simulink model "Lab_9_Electric_Power_Steering"  (R2023b)
settings: Solver=VariableStepAuto  StartTime=0.0  StopTime=20  RelTol=1e-3
libraries: fl_lib x20, nesl_utility x7, ee_lib x2, simulink x1
settings Model: Creator=AHMED MOHSEN  LastModifiedBy=AHMED MOHSEN

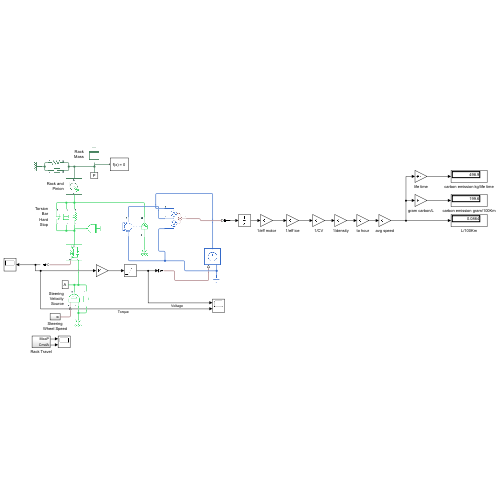
[thumbnail: Simulink's stored preview of the top-level diagram]
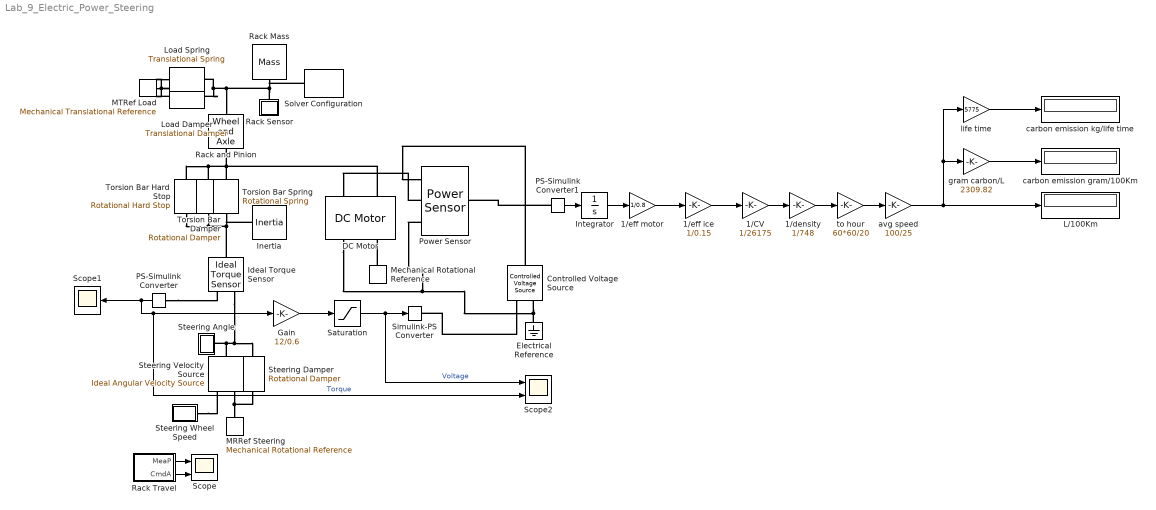
== system Lab_9_Electric_Power_Steering ==
  1/CV : Gain  Gain=1/26175
  1/density : Gain  Gain=1/748
  1/eff ice : Gain  Gain=1/0.15
  1/eff motor : Gain  Gain=1/0.8
  Controlled Voltage Source : fl_lib/Electrical/Electrical Sources/Controlled Voltage Source
  DC Motor : ee_lib/Electromechanical/Brushed Motors/DC Motor  field_option=ee.enum.field_option.pm  Rf=100 Ohm  Lf=1 H  Laf=0.15 H  If0=0 A  parameterization=ee.enum.dcparam_option.circuit_param  Ra=3.9 Ohm  La=12e-6 H  emf_or_torque=ee.enum.emf_or_torque.kv  Kv=0.072e-3 V/rpm  Ki=6.876e-4 N*m/A  T_stall=0.24e-3 N*m  w_max=19100 rpm  w_rated=15000 rpm  P_rated=0.08 W  V_rated=1.5 V  lam_param=ee.enum.lam_param.damping  i_noload=0 A  V_i_noload=1.5 V  J=0.01 cm^2*g  lam=0 N*m*s/rad  speed0=0 rpm  enable_fault_armature=simscape.enum.onoff.off  rev_faulted=1 / 3  G_faulted_armature=1e-5 S  fault_trigger_armature=ee.enum.faults.faultTrigger.temporal  t_fault_armature=1 s  max_permissible_current_armature=inf A  t_fail_on_current_armature=1 s  enable_fault_field=simscape.enum.onoff.off  G_faulted_field=1e-5 S  fault_trigger_field=ee.enum.faults.faultTrigger.temporal  t_fault_field=1 s  max_permissible_current_field=inf A  t_fail_on_current_field=1 s  fault_action=simscape.enum.assert.action.none  alpha=3.93e-3 1/K  Tmeas=25 degC  thermal_mass=100 J/K  initial_temperature=25 degC
  Electrical Reference : fl_lib/Electrical/Electrical Elements/Electrical Reference
  Gain : Gain  Gain=12/0.6
  Ideal Torque Sensor : fl_lib/Mechanical/Mechanical Sensors/Ideal Torque Sensor
  Inertia : fl_lib/Mechanical/Rotational Elements/Inertia  inertia=0.01 kg*m^2  num_ports=foundation.enum.numPorts2.one  w_specify=off  w_priority=High  w=0 rad/s  w_nominal_specify=off  w_nominal_unit=rad/s  w_nominal_value=1  t_specify=off  t_priority=None  t=0 N*m  t_nominal_specify=off  t_nominal_unit=N*m  t_nominal_value=1
  Integrator : Integrator
  L/100Km : Display
  Load Damper : fl_lib/Mechanical/Translational Elements/Translational Damper  Tag=Factory Generic  D=284 N/(m/s)  v_specify=off  v_priority=High  v=0 m/s  v_nominal_specify=off  v_nominal_unit=m/s  v_nominal_value=1  f_specify=off  f_priority=High  f=0 N  f_nominal_specify=off  f_nominal_unit=N  f_nominal_value=1
  Load Spring : fl_lib/Mechanical/Translational Elements/Translational Spring  Tag=Factory Generic  spr_rate=4450 N/m  v_specify=off  v_priority=High  v=0 m/s  v_nominal_specify=off  v_nominal_unit=m/s  v_nominal_value=1  f_specify=off  f_priority=High  f=0 N  f_nominal_specify=off  f_nominal_unit=N  f_nominal_value=1  x_specify=on  x_priority=High  x=0 m  x_nominal_specify=off  x_nominal_unit=m  x_nominal_value=1
  MRRef Steering : fl_lib/Mechanical/Rotational Elements/Mechanical Rotational Reference  Tag=Factory Generic
  MTRef Load : fl_lib/Mechanical/Translational Elements/Mechanical Translational Reference  Tag=Factory Generic
  Mechanical Rotational Reference : fl_lib/Mechanical/Rotational Elements/Mechanical Rotational Reference
  PS-Simulink Converter : nesl_utility/PS-Simulink Converter  PhysicalDomain=network_engine_domain  SubClassName=ps_output  LeftPortType=input  RightPortType=output  PseudoPeriodic=off  Frequencies=[]  VectorFormat=inherit  Unit=N*m  AffineConversion=off
  PS-Simulink Converter1 : nesl_utility/PS-Simulink Converter  PhysicalDomain=network_engine_domain  SubClassName=ps_output  LeftPortType=input  RightPortType=output  PseudoPeriodic=off  Frequencies=[]  VectorFormat=inherit  Unit=J/s  AffineConversion=off
  Power Sensor : ee_lib/Sensors & Transducers/Power Sensor  measurement_type=1  averaging_period=1e-4 s
  Rack Mass : fl_lib/Mechanical/Translational Elements/Mass  Tag=Factory Generic  mass=114 kg  num_ports=foundation.enum.numPorts2.one  v_specify=on  v_priority=High  v=0 m/s  v_nominal_specify=off  v_nominal_unit=m/s  v_nominal_value=1  f_specify=off  f_priority=High  f=0 N  f_nominal_specify=off  f_nominal_unit=N  f_nominal_value=1
  Rack Sensor : Subsystem
      mask Display: disp('P');
  Rack Travel : Subsystem
  Rack and Pinion : fl_lib/Mechanical/Mechanisms/Wheel and Axle  Tag=Factory Generic  R=3.8 cm  or=1  t_specify=off  t_priority=High  t=0 N*m  t_nominal_specify=off  t_nominal_unit=N*m  t_nominal_value=1  f_specify=off  f_priority=High  f=0 N  f_nominal_specify=off  f_nominal_unit=N  f_nominal_value=1
  Saturation : Saturate  UpperLimit=12  LowerLimit=-12
  Scope : Scope  NumInputPorts=2
  Scope1 : Scope
  Scope2 : Scope  NumInputPorts=2
  Simulink-PS Converter : nesl_utility/Simulink-PS Converter  PhysicalDomain=network_engine_domain  SubClassName=ps_input  LeftPortType=input  RightPortType=output  PseudoPeriodic=off  Frequencies=[]  NoiseDistribution=none  NoiseParameters=[]  Unit=V  AffineConversion=off  FilteringAndDerivatives=filter  SimscapeFilterOrder=1  InputFilterTimeConstant=0.001  UdotUserProvided=0
  Solver Configuration : nesl_utility/Solver Configuration  PhysicalDomain=network_engine_domain  SubClassName=solver  LeftPortType=input  RightPortType=generic  Tones=[]  Harmonics=[]  SimulateNoise=off  Profile=off  UseLocalSampling=off  EnableSwitchedLinearOptims=on  FrequencyDomain=off  UseCCode=off  RelTol=0.001  AbsTol=0.001  MinStep=1e-09  ToWorkspace=off  RevertToSquareIcSolve=off  NumHomotopyIterations=100  PhasorMode=off  PhasorModeNumHarmonics=1  ConsistencySolver=NEWTON_XTOL_AFTER_FTOL  IndexReductionMethod=DerivativeReplacement  DoDC=off  ResidualTolerance=1e-09  ConsistencyTolSource=GLOBAL  ConsistencyAbsTol=0.001  ConsistencyRelTol=0.001  ConsistencyTolFactor=0.001  UseLocalSolver=off  LocalSolverChoice=NE_BACKWARD_EULER_ADVANCER  ResolveIndetEquations=on  FunctionEvalNumThread=1  LocalSolverSampleTime=0.001  DoFixedCost=off  MaxNonlinIter=3  MaxModeIter=2  ComputeImpulses=off  ImpulseIterations=2  LinearAlgebra=auto  LinearAlgebraNumThread=0  EquationFormulation=NE_TIME_EF  DelaysMemoryBudget=1024  AutomaticFiltering=on  FilteringTimeConstant=0.001  PartitionStorageMethod=AS_NEEDED  PartitionMemoryBudget=1024  PartitionMethod=ROBUST  MultibodyUseLocalSolver=off  MultibodyLocalSolverChoice=ODE1  MultibodyLocalSolverSampleTime=0.001
  Steering Angle : Subsystem
      mask Display: disp('A');
  Steering Damper : fl_lib/Mechanical/Rotational Elements/Rotational Damper  Tag=Factory Generic  D=0.001 N*m/(rad/s)  w_specify=off  w_priority=High  w=0 rad/s  w_nominal_specify=off  w_nominal_unit=rad/s  w_nominal_value=1  t_specify=off  t_priority=High  t=0 N*m  t_nominal_specify=off  t_nominal_unit=N*m  t_nominal_value=1
  Steering Velocity Source : fl_lib/Mechanical/Mechanical Sources/Ideal Angular Velocity Source  Tag=Factory Generic
  Steering Wheel Speed : Subsystem
  Torsion Bar Hard Stop : fl_lib/Mechanical/Rotational Elements/Rotational Hard Stop  Tag=Factory Generic  upper_bnd=9 deg  lower_bnd=-9 deg  model=3  stiff_up=1e+06 N*m/rad  stiff_low=1e6 N*m/rad  D_up=0.01 N*m/(rad/s)  D_low=0.01 N*m/(rad/s)  transition=0.001 rad  coeff_rest=0.7  w_tol=0.1 rad/s  trq_tol=0.001 N*m  w_specify=off  w_priority=High  w=0 rad/s  w_nominal_specify=off  w_nominal_unit=rad/s  w_nominal_value=1  t_specify=off  t_priority=High  t=0 N*m  t_nominal_specify=off  t_nominal_unit=N*m  t_nominal_value=1  phi_specify=on  phi_priority=High  phi=0 rad  phi_nominal_specify=off  phi_nominal_unit=rad  phi_nominal_value=1  M_specify=off  M_priority=None  M=0
  Torsion Bar Damper : fl_lib/Mechanical/Rotational Elements/Rotational Damper  Tag=Factory Generic  D=0.01 N*m/(rad/s)  w_specify=off  w_priority=High  w=0 rad/s  w_nominal_specify=off  w_nominal_unit=rad/s  w_nominal_value=1  t_specify=off  t_priority=High  t=0 N*m  t_nominal_specify=off  t_nominal_unit=N*m  t_nominal_value=1
  Torsion Bar Spring : fl_lib/Mechanical/Rotational Elements/Rotational Spring  Tag=Factory Generic  spr_rate=10 N*m/rad  w_specify=off  w_priority=High  w=0 rad/s  w_nominal_specify=off  w_nominal_unit=rad/s  w_nominal_value=1  t_specify=off  t_priority=High  t=0 N*m  t_nominal_specify=off  t_nominal_unit=N*m  t_nominal_value=1  phi_specify=on  phi_priority=High  phi=0 rad  phi_nominal_specify=off  phi_nominal_unit=rad  phi_nominal_value=1
  avg speed : Gain  Gain=100/25
  carbon emission gram/100Km : Display
  carbon emission kg/life time : Display
  gram carbon/L : Gain  Gain=2309.82
  life time : Gain  Gain=5775
  to hour : Gain  Gain=60*60/20
  wires:
  Rack Travel/2(CmdA) -> Scope/2
  Rack Travel/1(MeaP) -> Scope/1
  PS-Simulink Converter/1 -> Gain/1, Scope2/2, Scope1/1  "Torque"
  Gain/1 -> Saturation/1
  Saturation/1 -> Scope2/1, Simulink-PS Converter/1  "Voltage"
  PS-Simulink Converter1/1 -> Integrator/1
  Integrator/1 -> 1/eff motor/1
  1/eff motor/1 -> 1/eff ice/1
  1/eff ice/1 -> 1/CV/1
  1/CV/1 -> 1/density/1
  1/density/1 -> to hour/1
  to hour/1 -> avg speed/1
  avg speed/1 -> life time/1, gram carbon/L/1, L/100Km/1
  gram carbon/L/1 -> carbon emission gram/100Km/1
  life time/1 -> carbon emission kg/life time/1
  connections:
  Torsion Bar Spring/LConn1 -- DC Motor/LConn2 -- Rack and Pinion/LConn1 -- Torsion Bar Hard Stop/LConn1 -- Torsion Bar Damper/LConn1
  Load Spring/RConn1 -- MTRef Load/LConn1 -- Load Damper/RConn1
  Load Damper/LConn1 -- Solver Configuration/RConn1 -- Rack Mass/LConn1 -- Rack Sensor/LConn1 -- Rack and Pinion/RConn1 -- Load Spring/LConn1
  MRRef Steering/LConn1 -- Steering Velocity Source/RConn2 -- Steering Damper/RConn1
  Steering Angle/LConn1 -- Ideal Torque Sensor/RConn1 -- Steering Damper/LConn1 -- Steering Velocity Source/LConn1
  Steering Wheel Speed/RConn1 -- Steering Velocity Source/RConn1
  Torsion Bar Hard Stop/RConn1 -- Torsion Bar Damper/RConn1 -- Ideal Torque Sensor/LConn1 -- Inertia/LConn1 -- Torsion Bar Spring/RConn1
  PS-Simulink Converter/LConn1 -- Ideal Torque Sensor/RConn2
  Mechanical Rotational Reference/LConn1 -- DC Motor/RConn2
  Controlled Voltage Source/RConn1 -- Simulink-PS Converter/RConn1
  Electrical Reference/LConn1 -- Power Sensor/LConn3 -- DC Motor/RConn1 -- Controlled Voltage Source/RConn2
  Controlled Voltage Source/LConn1 -- Power Sensor/LConn1
  Power Sensor/LConn2 -- DC Motor/LConn1
  PS-Simulink Converter1/LConn1 -- Power Sensor/RConn1

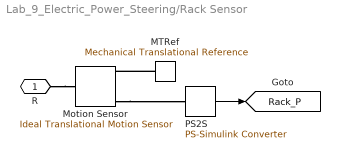
== system Lab_9_Electric_Power_Steering/Rack Sensor ==
  MTRef : fl_lib/Mechanical/Translational Elements/Mechanical Translational Reference  Tag=Factory Generic
  Motion Sensor : fl_lib/Mechanical/Mechanical Sensors/Ideal Translational Motion Sensor  Tag=Factory Generic  reference=foundation.enum.MeasurementReference.difference  acceleration_port=false  velocity_port=true  position_port=true  offset=0 m
  PS2S : nesl_utility/PS-Simulink Converter  PhysicalDomain=network_engine_domain  SubClassName=ps_output  LeftPortType=input  RightPortType=output  PseudoPeriodic=off  Frequencies=[]  VectorFormat=1-D array  Unit=m  AffineConversion=off
  R : PMIOPort  Side=Left
  tag scope: Rack_P=global
  wires:
  PS2S/1 -> [Rack_P]
  connections:
  R/RConn1 -- Motion Sensor/LConn1
  Motion Sensor/RConn3 -- PS2S/LConn1
  MTRef/LConn1 -- Motion Sensor/RConn1

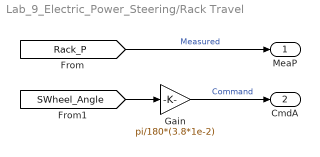
== system Lab_9_Electric_Power_Steering/Rack Travel ==
  Gain : Gain  Gain=pi/180*(3.8*1e-2)
  MeaP : Outport  VectorParamsAs1DForOutWhenUnconnected=off
  CmdA : Outport  Port=2  VectorParamsAs1DForOutWhenUnconnected=off
  wires:
  [Rack_P] -> MeaP/1  "Measured"
  [SWheel_Angle] -> Gain/1
  Gain/1 -> CmdA/1  "Command"

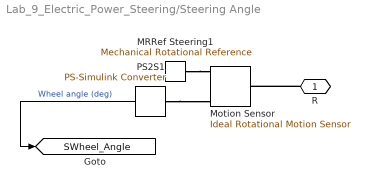
== system Lab_9_Electric_Power_Steering/Steering Angle ==
  MRRef Steering1 : fl_lib/Mechanical/Rotational Elements/Mechanical Rotational Reference  Tag=Factory Generic
  Motion Sensor : fl_lib/Mechanical/Mechanical Sensors/Ideal Rotational Motion Sensor  Tag=Factory Generic  reference=foundation.enum.MeasurementReference.difference  acceleration_port=false  velocity_port=true  position_port=true  wrap_angle=simscape.enum.onoff.off  offset=0 rad
  PS2S1 : nesl_utility/PS-Simulink Converter  PhysicalDomain=network_engine_domain  SubClassName=ps_output  LeftPortType=input  RightPortType=output  PseudoPeriodic=off  Frequencies=[]  VectorFormat=1-D array  Unit=deg  AffineConversion=off
  R : PMIOPort  Side=Left
  tag scope: SWheel_Angle=global
  wires:
  PS2S1/1 -> [SWheel_Angle]  "Wheel angle (deg)"
  connections:
  PS2S1/LConn1 -- Motion Sensor/RConn3
  R/RConn1 -- Motion Sensor/LConn1
  MRRef Steering1/LConn1 -- Motion Sensor/RConn1

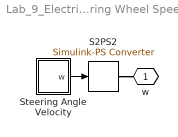
== system Lab_9_Electric_Power_Steering/Steering Wheel Speed ==
  S2PS2 : nesl_utility/Simulink-PS Converter  PhysicalDomain=network_engine_domain  SubClassName=ps_input  LeftPortType=input  RightPortType=output  PseudoPeriodic=off  Frequencies=[]  NoiseDistribution=none  NoiseParameters=[]  Unit=rpm  AffineConversion=off  FilteringAndDerivatives=filter  SimscapeFilterOrder=1  InputFilterTimeConstant=.001  UdotUserProvided=0
  Steering Angle Velocity : Subsystem
  w : PMIOPort  Side=Right
  wires:
  Steering Angle Velocity/1(w) -> S2PS2/1
  connections:
  S2PS2/RConn1 -- w/RConn1

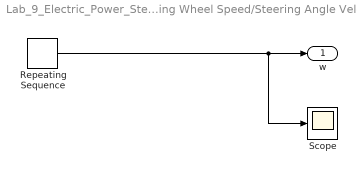
== system Lab_9_Electric_Power_Steering/Steering Wheel Speed/Steering Angle Velocity ==
  Repeating Sequence : simulink/Sources/Repeating Sequence  rep_seq_t=[0 1.96 2.4 4.05 4.5 5.95 6.75 8.05 8.4 10 10.35 11.7 12 13.85 14.2 15.7 15.95 20]  rep_seq_y=[0 0 0.99 1 0 0 -1 -1 0 0 -1 -0.99 0 0 1 1 0 0]
  Scope : Scope
  w : Outport
  wires:
  Repeating Sequence/1 -> Scope/1, w/1
